simulink subsystem "Gearbox_Ver1"  (R2023a)
settings: Solver=VariableStepAuto  StartTime=0.0  StopTime=10.0  RelTol=1e-3
undefined symbols (not defined in the file or in its folder): a, c, F2, G2, i, Jn
settings Model: Creator=ycheb  LastModifiedBy=ycheb

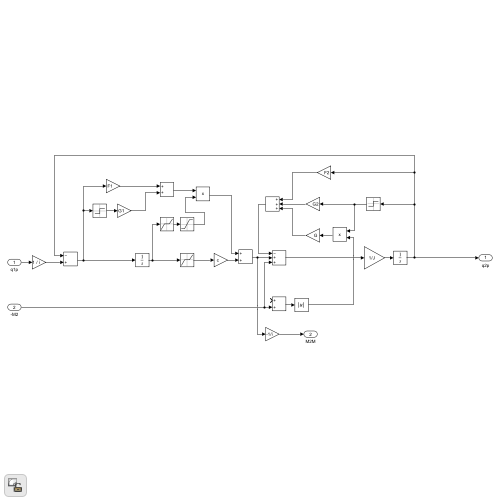
[thumbnail: Simulink's stored preview of the top-level diagram]
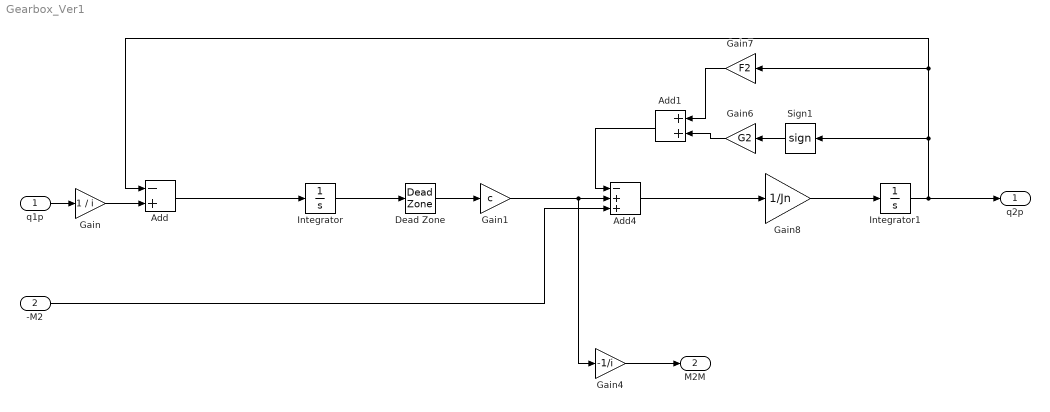
== system Gearbox_Ver1 ==
  q1p : Inport
  -M2 : Inport  Port=2
  Add : Sum  Inputs=-+
  Add1 : Sum
  Add4 : Sum  Inputs=-++
  Dead Zone : DeadZone  LowerValue=-a  UpperValue=a
  Gain : Gain  Gain=1 / i
  Gain1 : Gain  Gain=c
  Gain4 : Gain  Gain=-1/i
  Gain6 : Gain  Gain=G2
  Gain7 : Gain  Gain=F2
  Gain8 : Gain  Gain=1/Jn
  Integrator : Integrator
  Integrator1 : Integrator
  Sign1 : Signum
  q2p : Outport
  M2M : Outport  Port=2
  wires:
  q1p/1 -> Gain/1
  Gain/1 -> Add/2
  Add/1 -> Integrator/1
  Integrator/1 -> Dead Zone/1
  Dead Zone/1 -> Gain1/1
  -M2/1 -> Add4/3
  Gain1/1 -> Gain4/1, Add4/2
  Gain4/1 -> M2M/1
  Add4/1 -> Gain8/1
  Gain8/1 -> Integrator1/1
  Integrator1/1 -> q2p/1, Sign1/1, Gain7/1, Add/1
  Gain7/1 -> Add1/1
  Sign1/1 -> Gain6/1
  Gain6/1 -> Add1/2
  Add1/1 -> Add4/1
